simulink model "Diagrama_nanofiltracion"  (R2019a)
settings: Solver=VariableStepAuto  StartTime=0.0  StopTime=24.0  RelTol=1e-3
libraries: Libreria x6
settings Model: Creator=Usuario  LastModifiedBy=Usuario

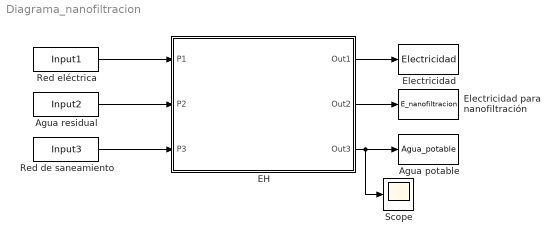
== system Diagrama_nanofiltracion ==
  Agua potable : ToWorkspace  VariableName=Agua_potable  SaveFormat=Timeseries  SampleTime=-1
  Agua residual : FromWorkspace  VariableName=Input2  SampleTime=0
  EH : Subsystem
  Electricidad : ToWorkspace  VariableName=Electricidad  SaveFormat=Timeseries  SampleTime=-1
  Electricidad para nanofiltración : ToWorkspace  VariableName=E_nanofiltracion  SaveFormat=Timeseries  SampleTime=-1
  Red de saneamiento : FromWorkspace  VariableName=Input3  SampleTime=0
  Red eléctrica : FromWorkspace  VariableName=Input1  SampleTime=0
  Scope : Scope
  wires:
  Red eléctrica/1 -> EH/1(P1)
  Agua residual/1 -> EH/2(P2)
  Red de saneamiento/1 -> EH/3(P3)
  EH/1(Out1) -> Electricidad/1
  EH/2(Out2) -> Electricidad para nanofiltración/1
  EH/3(Out3) -> Scope/1, Agua potable/1

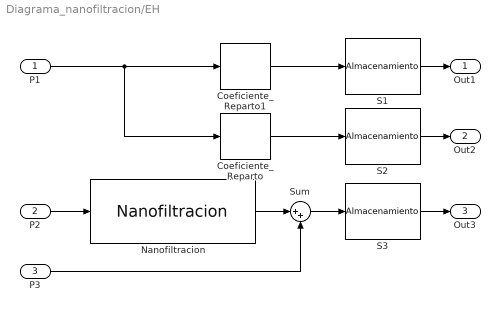
== system Diagrama_nanofiltracion/EH ==
  P1 : Inport
  P2 : Inport  Port=2
  P3 : Inport  Port=3
  Coeficiente_Reparto : Libreria/Coeficiente_Reparto  dispatch_factor=alfa2  Tm=T_muestreo  Max_out=inf  Max_in=inf  efficiency=1
  Coeficiente_Reparto1 : Libreria/Coeficiente_Reparto  dispatch_factor=alfa1  Tm=T_muestreo  Max_out=inf  Max_in=inf  efficiency=1
  Nanofiltracion : Libreria/Nanofiltracion  efficiency=0.95  dispatch_factor=beta1  T_muestreo=T_muestreo  Max_in=60  Max_out=60  n_salida=[2]
  S1 : Libreria/Almacenamiento  Up2=1  Low2=0  r_c=1  Up=1  Low=0  r_d=1  Up1=10  Low1=0  almacenamiento_inicial=0  cpa=1  almacenamiento_on=off
      link override In1: SampleTime=1
      link override Qch: VariableName=Qchp1
      link override Qdis: VariableName=Qdisp1
      link override almacenamiento: VariableName=almacen1
      link override discrepancias_almacenamiento: VariableName=discrepancias_almacenamiento1
      link override ef: VariableName=Ech1
      link override eff: VariableName=Edis1
  S2 : Libreria/Almacenamiento  Up2=1  Low2=0  r_c=1  Up=1  Low=0  r_d=1  Up1=4  Low1=0  almacenamiento_inicial=0  cpa=1  almacenamiento_on=off
      link override In1: SampleTime=1
      link override Qch: VariableName=Qchp2
      link override Qdis: VariableName=Qdisp2
      link override almacenamiento: VariableName=almacen2
      link override discrepancias_almacenamiento: VariableName=discrepancias_almacenamiento2
      link override ef: VariableName=Ech2
      link override eff: VariableName=Edis2
  S3 : Libreria/Almacenamiento  Up2=80  Low2=0  r_c=1  Up=80  Low=0  r_d=1  Up1=250  Low1=0  almacenamiento_inicial=0  cpa=1  almacenamiento_on=on
      link override In1: SampleTime=1
      link override Qch: VariableName=Qchp3
      link override Qdis: VariableName=Qdisp3
      link override almacenamiento: VariableName=almacen3
      link override discrepancias_almacenamiento: VariableName=discrepancias_almacenamiento3
      link override ef: VariableName=Ech3
      link override eff: VariableName=Edis3
  Sum : Sum  Inputs=|++
  Out1 : Outport
  Out2 : Outport  Port=2
  Out3 : Outport  Port=3
  wires:
  S3/1 -> Out3/1
  Coeficiente_Reparto1/1 -> S1/1
  P1/1 -> Coeficiente_Reparto/1, Coeficiente_Reparto1/1
  Coeficiente_Reparto/1 -> S2/1
  S1/1 -> Out1/1
  S2/1 -> Out2/1
  P2/1 -> Nanofiltracion/1
  Sum/1 -> S3/1
  Nanofiltracion/1 -> Sum/1
  P3/1 -> Sum/2
